simulink model "3Zad_Adasiak"  (R2020b)
settings: Solver=VariableStepAuto  StartTime=0.0  StopTime=0.0  RelTol=1e-3
undefined symbols (not defined in the file): W
libraries: CPOiS_SourcesSinks x24, CPOiS_DataManipulation_DataTypeConversion x12, CPOiS_LinearTransforms x8, CPOiS_Filters x4, CPOiS_General x1
settings Model: Creator=Krystian  LastModifiedBy=Krystian

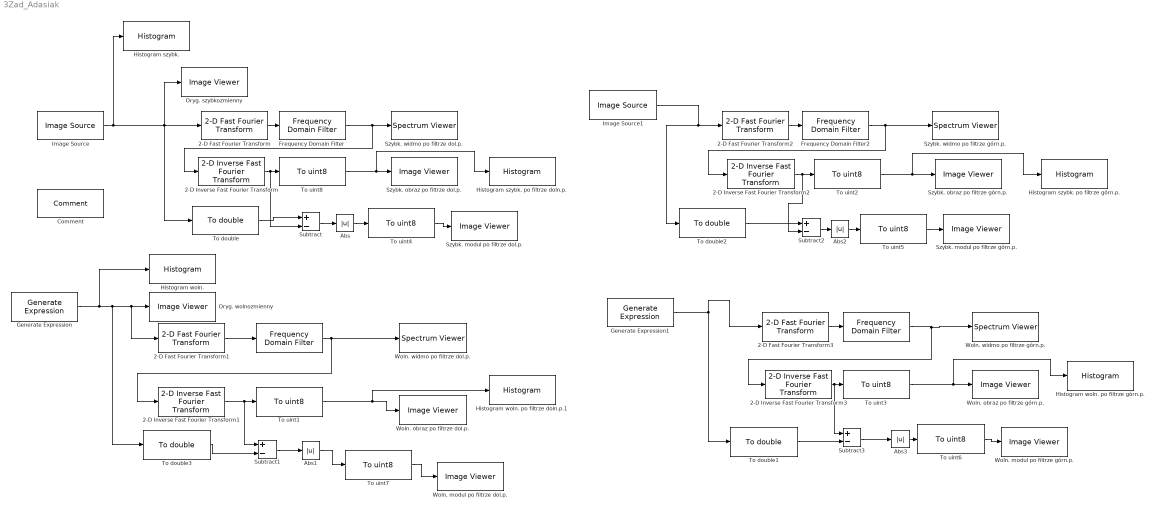
== system 3Zad_Adasiak ==
  " " : CPOiS_Filters/Frequency Domain Filter  filtertype=High-pass Filter  radius=10
      settings: SourceProductName=CPOiS - Digital image and signal processing
  "  " : CPOiS_Filters/Frequency Domain Filter  filtertype=Low-pass Filter  radius=10
      settings: SourceProductName=CPOiS - Digital image and signal processing
  2-D Fast Fourier Transform{,1..3} (4 alike) : CPOiS_LinearTransforms/2-D Fast Fourier Transform
      settings: SourceProductName=CPOiS - Digital image and signal processing
  2-D Inverse Fast Fourier Transform{,1..3} (4 alike) : CPOiS_LinearTransforms/2-D Inverse Fast  Fourier Transform
      settings: SourceProductName=CPOiS - Digital image and signal processing
  Abs{,1..3} (4 alike) : Abs
  Comment : CPOiS_General/Comment
      settings: SourceProductName=CPOiS - Digital image and signal processing
  Frequency Domain Filter : CPOiS_Filters/Frequency Domain Filter  filtertype=Low-pass Filter  radius=10
      settings: SourceProductName=CPOiS - Digital image and signal processing
  Frequency Domain Filter2 : CPOiS_Filters/Frequency Domain Filter  filtertype=High-pass Filter  radius=10
      settings: SourceProductName=CPOiS - Digital image and signal processing
  Generate Expression : CPOiS_SourcesSinks/Generate Expression  Width=256  Height=256  Expression=128.*(sin(W)+1)
      settings: SourceProductName=CPOiS - Digital image and signal processing
  Generate Expression1 : CPOiS_SourcesSinks/Generate Expression  Width=256  Height=256  Expression=128.*(sin(W)+1)
      settings: SourceProductName=CPOiS - Digital image and signal processing
  Histogram szybk. : CPOiS_SourcesSinks/Histogram
      settings: SourceProductName=CPOiS - Digital image and signal processing
  Histogram szybk. po filtrze doln.p. : CPOiS_SourcesSinks/Histogram
      settings: SourceProductName=CPOiS - Digital image and signal processing
  Histogram szybk. po filtrze górn.p. : CPOiS_SourcesSinks/Histogram
      settings: SourceProductName=CPOiS - Digital image and signal processing
  Histogram woln. : CPOiS_SourcesSinks/Histogram
      settings: SourceProductName=CPOiS - Digital image and signal processing
  Histogram woln. po filtrze doln.p.1 : CPOiS_SourcesSinks/Histogram
      settings: SourceProductName=CPOiS - Digital image and signal processing
  Histogram woln. po filtrze górn.p. : CPOiS_SourcesSinks/Histogram
      settings: SourceProductName=CPOiS - Digital image and signal processing
  Image Source : CPOiS_SourcesSinks/Image Source  FileSelection=moon.png
      settings: SourceProductName=CPOiS - Digital image and signal processing
  Image Source1 : CPOiS_SourcesSinks/Image Source  FileSelection=moon.png
      settings: SourceProductName=CPOiS - Digital image and signal processing
  Oryg. szybkozmienny : CPOiS_SourcesSinks/Image Viewer
      settings: SourceProductName=CPOiS - Digital image and signal processing
  Oryg. wolnozmienny : CPOiS_SourcesSinks/Image Viewer
      settings: SourceProductName=CPOiS - Digital image and signal processing
  Subtract{,1..3} (4 alike) : Sum  Inputs=+-
  Szybk. modul po filtrze dol.p. : CPOiS_SourcesSinks/Image Viewer
      settings: SourceProductName=CPOiS - Digital image and signal processing
  Szybk. modul po filtrze górn.p. : CPOiS_SourcesSinks/Image Viewer
      settings: SourceProductName=CPOiS - Digital image and signal processing
  Szybk. obraz po filtrze dol.p. : CPOiS_SourcesSinks/Image Viewer
      settings: SourceProductName=CPOiS - Digital image and signal processing
  Szybk. obraz po filtrze górn.p. : CPOiS_SourcesSinks/Image Viewer
      settings: SourceProductName=CPOiS - Digital image and signal processing
  Szybk. widmo po filtrze dol.p. : CPOiS_SourcesSinks/Spectrum Viewer
      settings: SourceProductName=CPOiS - Digital image and signal processing
  Szybk. widmo po filtrze górn.p. : CPOiS_SourcesSinks/Spectrum Viewer
      settings: SourceProductName=CPOiS - Digital image and signal processing
  To double{,1..3} (4 alike) : CPOiS_DataManipulation_DataTypeConversion/To double
      settings: SourceProductName=CPOiS - Digital image and signal processing
  To uint{1..8} (8 alike) : CPOiS_DataManipulation_DataTypeConversion/To uint8
      settings: SourceProductName=CPOiS - Digital image and signal processing
  Woln. modul po filtrze dol.p. : CPOiS_SourcesSinks/Image Viewer
      settings: SourceProductName=CPOiS - Digital image and signal processing
  Woln. modul po filtrze górn.p. : CPOiS_SourcesSinks/Image Viewer
      settings: SourceProductName=CPOiS - Digital image and signal processing
  Woln. obraz po filtrze dol.p. : CPOiS_SourcesSinks/Image Viewer
      settings: SourceProductName=CPOiS - Digital image and signal processing
  Woln. obraz po filtrze górn.p. : CPOiS_SourcesSinks/Image Viewer
      settings: SourceProductName=CPOiS - Digital image and signal processing
  Woln. widmo po filtrze dol.p. : CPOiS_SourcesSinks/Spectrum Viewer
      settings: SourceProductName=CPOiS - Digital image and signal processing
  Woln. widmo po filtrze górn.p. : CPOiS_SourcesSinks/Spectrum Viewer
      settings: SourceProductName=CPOiS - Digital image and signal processing
  wires:
  2-D Fast Fourier Transform2/1 -> Frequency Domain Filter2/1
  Image Source1/1 -> To double2/1, 2-D Fast Fourier Transform2/1
  Subtract3/1 -> Abs3/1
  To uint1/1 -> Histogram woln. po filtrze doln.p.1/1, Woln. obraz po filtrze dol.p./1
  2-D Fast Fourier Transform/1 -> Frequency Domain Filter/1
  2-D Inverse Fast Fourier Transform3/1 -> Subtract3/1, To uint3/1
  To uint2/1 -> Histogram szybk. po filtrze górn.p./1, Szybk. obraz po filtrze górn.p./1
  To uint3/1 -> Histogram woln. po filtrze górn.p./1, Woln. obraz po filtrze górn.p./1
  "  "/1 -> 2-D Inverse Fast Fourier Transform1/1, Woln. widmo po filtrze dol.p./1
  " "/1 -> 2-D Inverse Fast Fourier Transform3/1, Woln. widmo po filtrze górn.p./1
  2-D Fast Fourier Transform3/1 -> " "/1
  Frequency Domain Filter2/1 -> Szybk. widmo po filtrze górn.p./1, 2-D Inverse Fast Fourier Transform2/1
  Frequency Domain Filter/1 -> 2-D Inverse Fast Fourier Transform/1, Szybk. widmo po filtrze dol.p./1
  Generate Expression1/1 -> 2-D Fast Fourier Transform3/1, To double1/1
  Subtract/1 -> Abs/1
  Image Source/1 -> To double/1, 2-D Fast Fourier Transform/1, Oryg. szybkozmienny/1, Histogram szybk./1
  To uint8/1 -> Histogram szybk. po filtrze doln.p./1, Szybk. obraz po filtrze dol.p./1
  2-D Inverse Fast Fourier Transform2/1 -> Subtract2/2, To uint2/1
  Subtract2/1 -> Abs2/1
  2-D Fast Fourier Transform1/1 -> "  "/1
  Subtract1/1 -> Abs1/1
  Generate Expression/1 -> Histogram woln./1, Oryg. wolnozmienny/1, 2-D Fast Fourier Transform1/1, To double3/1
  2-D Inverse Fast Fourier Transform1/1 -> Subtract1/1, To uint1/1
  2-D Inverse Fast Fourier Transform/1 -> Subtract/2, To uint8/1
  To double/1 -> Subtract/1
  To double1/1 -> Subtract3/2
  To double3/1 -> Subtract1/2
  To double2/1 -> Subtract2/1
  Abs/1 -> To uint4/1
  To uint4/1 -> Szybk. modul po filtrze dol.p./1
  Abs2/1 -> To uint5/1
  To uint5/1 -> Szybk. modul po filtrze górn.p./1
  Abs3/1 -> To uint6/1
  To uint6/1 -> Woln. modul po filtrze górn.p./1
  To uint7/1 -> Woln. modul po filtrze dol.p./1
  Abs1/1 -> To uint7/1
